simulink model "rocket"  (R2024a)
settings: Solver=ode5  StartTime=0.0  StopTime=time  FixedStep=0.01  RelTol=1e-3
values from neighbouring files (symbols this model uses):
  angle_ref = 0    [main.m]
  dt = 4    [main.m]
  F_side_thruster = 440    [main.m]
  F_thruster = 111000    [main.m]
  g = 9.81    [main.m]
  height = 8.15    [main.m]
  J = 1/12*m *(height^2 + 3*radius^2)    (= 4215.95433333)    [main.m]
  k = 0.02    [main.m]
  Ka = 1    [main.m]
  Kd = 0    [main.m]
  Ki = 0    [main.m]
  Kp = 0    [main.m]
  m = 760    [main.m]
  radius = 0.22    [main.m]
undefined symbols (not defined in the file or in its folder): W
settings Model: Creator=erlin  LastModifiedBy=erlin

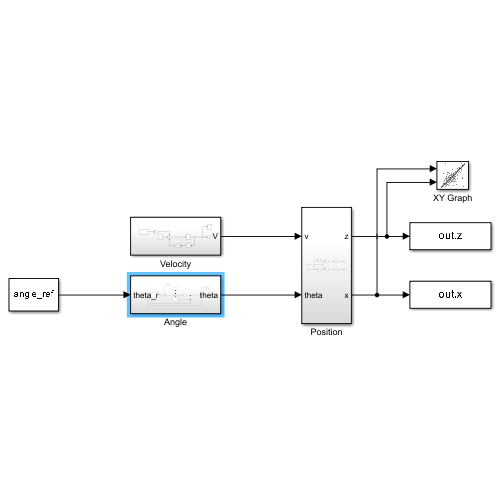
[thumbnail: Simulink's stored preview of the top-level diagram]
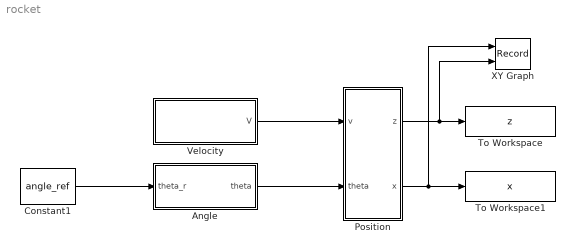
== system rocket ==
  Angle : Subsystem
  Constant1 : Constant  Value=angle_ref
  Position : Subsystem
  To Workspace : ToWorkspace  VariableName=z  SaveFormat=Timeseries  SampleTime=-1
  To Workspace1 : ToWorkspace  VariableName=x  SaveFormat=Timeseries  SampleTime=-1
  Velocity : Subsystem
  XY Graph : Record  FileSettingsInternal="{\"entries\":[{\"content\":{\"excelSettings\":{\"content\":{},\"type\":\"Streamout.ExcelSettings\"}},\"type\":\"Streamout.FileSettingStorage\",\"uuid\":\"\"}],\"packageUris\":[\"http:\\/\\/schema.mathworks.com\\/mf0\\/streamout_blocks\\/R2020a\"],\"version\":\"1.0\"}"  Layout=[1 1]  SignalsInternal="{\"entries\":[{\"content\":{\"signals\":[{\"content\":{\"blockPath\":[],\"dimensions\":[1],\"domain\":\"\",\"lineColor\":\"#a2142f\",\"plots\":[ 1 ],\"port\":1,\"sid\":[\"\"],\"signalID\":1,\"signalName\":\"Position:2\"},\"type\":\"RecordBlkView.Signal\",\"uuid\":\"\"},{\"content\":{\"blockPath\":[],\"dimensions\":[1],\"domain\":\"\",\"lineColor\":\"#139fff\",\"plots\":[ 1 ],\"port\":2,\"sid\":[\"\"],\"signalID\":2,\"signalName\":\"Position:1\"},\"type\":\"RecordBlkView.Signal\",\"uuid\":\"\"}]},\"type\":\"RecordBlkView.InputSignals\",\"uuid\":\"\"}],\"packageUris\":[\"http:\\/\\/schema.mathworks.com\\/mf0\\/streamout_blocks\\/R2020a\"],\"version\":\"1.0\"}"  VisualizationBindings="{\"xyplotplugin\":{\"info\":[{\"series\":[{\"bindingParametersList\":[{\"parameter\":\"X-Axis\",\"signalID\":1,\"signalName\":\"Position:2\"},{\"parameter\":\"Y-Axis\",\"signalID\":2,\"signalName\":\"Position:1\"}],\"seriesID\":0}],\"subplotID\":1}]}}"  CompatibilityTag=XY
  wires:
  Velocity/1(V) -> Position/1(v)
  Angle/1(theta) -> Position/2(theta)
  Position/1(z) -> XY Graph/2, To Workspace/1
  Position/2(x) -> XY Graph/1, To Workspace1/1
  Constant1/1 -> Angle/1(theta_r)

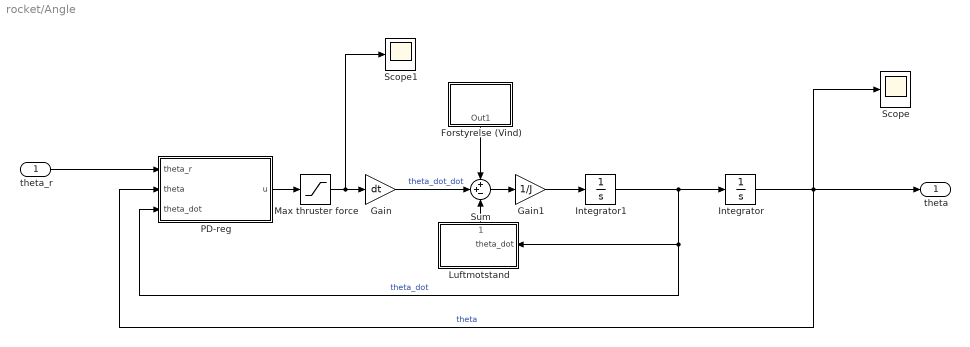
== system rocket/Angle ==
  theta_r : Inport
  Forstyrelse (Vind) : Subsystem
  Gain : Gain  Gain=dt
  Gain1 : Gain  Gain=1/J
  Integrator : Integrator
  Integrator1 : Integrator
  Luftmotstand : Subsystem
      settings: PortSchema="{\"entries\":[{\"content\":{\"sides\":[{\"content\":{},\"type\":\"ConnectorPlacement.EquallySpacedRectSide\",\"uuid\":\"0698149c-fc66-40d5-96ad-7619179b653e\"},{\"content\":{\"connectorIds\":[\"Out1\"],\"side\":\"RIGHT\"},\"type\":\"ConnectorPlacement.EquallySpacedRectSide\",\"uuid\":\"7770e965-7410-4cbf-a102-79b4cde0d90a\"},{\"content\":{\"side\":\"TOP\"},\"type\":\"ConnectorPlacement.EquallySpacedRectSide\",\"uuid\":\"2756d427-3d7a-4b20-bd26-ca223827eea1\"},{\"content\":{\"connectorIds\":[\"In1\"],\"side\":\"BOTTOM\"},\"type\":\"ConnectorPlacement.EquallySpacedRectSide\",\"uuid\":\"1c0a4e01-980e-4eae-bcaf-d8b95709db4d\"}]},\"type\":\"ConnectorPlacement.EquallySpacedConnector\",\"uuid\":\"871502e0-b275-4b38-8496-5b51979ecd95\"}],\"packageUris\":[\"http://schema.mathworks.com/mf0/Connector/R2020b\"],\"version\":\"1.0\"}"
  Max thruster force : Saturate  UpperLimit=F_side_thruster  LowerLimit=-F_side_thruster
  PD-reg : Subsystem
  Scope : Scope
  Scope1 : Scope
  Sum : Sum  Inputs=++-
  theta : Outport
  wires:
  Integrator1/1 -> Integrator/1, PD-reg/3(theta_dot), Luftmotstand/1(theta_dot)  "theta_dot"
  Integrator/1 -> PD-reg/2(theta), theta/1, Scope/1  "theta"
  Sum/1 -> Gain1/1
  Gain/1 -> Sum/2  "theta_dot_dot"
  theta_r/1 -> PD-reg/1(theta_r)
  Forstyrelse (Vind)/1(Out1) -> Sum/1
  PD-reg/1(u) -> Max thruster force/1
  Luftmotstand/1(1) -> Sum/3
  Gain1/1 -> Integrator1/1
  Max thruster force/1 -> Scope1/1, Gain/1

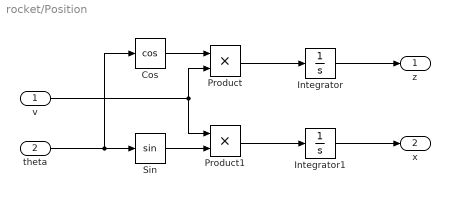
== system rocket/Position ==
  v : Inport
  theta : Inport  Port=2
  Cos : Trigonometry  Operator=cos
  Integrator : Integrator
  Integrator1 : Integrator
  Product : Product
  Product1 : Product
  Sin : Trigonometry
  z : Outport
  x : Outport  Port=2
  wires:
  theta/1 -> Cos/1, Sin/1
  v/1 -> Product1/1, Product/2
  Product/1 -> Integrator/1
  Product1/1 -> Integrator1/1
  Sin/1 -> Product1/2
  Integrator/1 -> z/1
  Integrator1/1 -> x/1
  Cos/1 -> Product/1

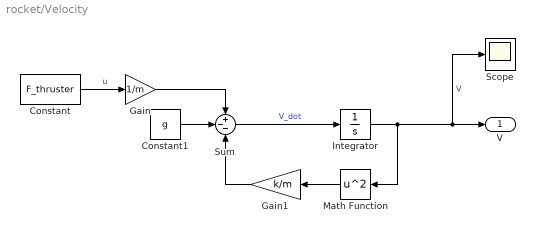
== system rocket/Velocity ==
  Constant : Constant  Value=F_thruster
  Constant1 : Constant  Value=g
  Gain : Gain  Gain=1/m
  Gain1 : Gain  Gain=k/m
  Integrator : Integrator
  Math Function : Math  Operator=square
  Scope : Scope
  Sum : Sum  Inputs=+--
  V : Outport
  wires:
  Constant1/1 -> Sum/2
  Gain/1 -> Sum/1
  Gain1/1 -> Sum/3
  Constant/1 -> Gain/1  "u"
  Integrator/1 -> Math Function/1, Scope/1, V/1  "V"
  Math Function/1 -> Gain1/1
  Sum/1 -> Integrator/1  "V_dot"

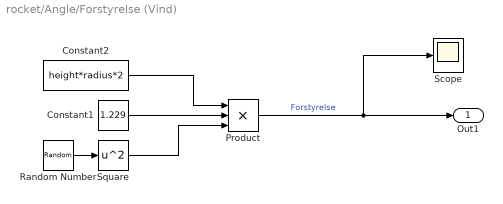
== system rocket/Angle/Forstyrelse (Vind) ==
  Constant1 : Constant  Value=1.229
  Constant2 : Constant  Value=height*radius*2
  Product : Product  Inputs=3
  Random Number : RandomNumber  Mean=W  Variance=W/2  SampleTime=10
  Scope : Scope
  Square : Math  Operator=square
  Out1 : Outport
  wires:
  Product/1 -> Scope/1, Out1/1  "Forstyrelse"
  Constant1/1 -> Product/2
  Constant2/1 -> Product/1
  Random Number/1 -> Square/1
  Square/1 -> Product/3

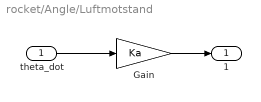
== system rocket/Angle/Luftmotstand ==
  theta_dot : Inport
  Gain : Gain  Gain=Ka
  1 : Outport
  wires:
  Gain/1 -> 1/1
  theta_dot/1 -> Gain/1

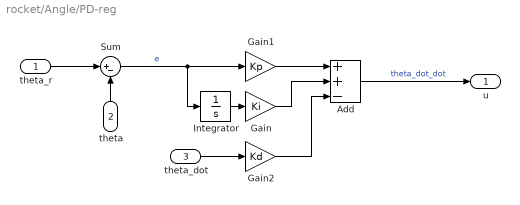
== system rocket/Angle/PD-reg ==
  theta_r : Inport
  theta : Inport  Port=2
  theta_dot : Inport  Port=3
  Add : Sum  Inputs=++-
  Gain : Gain  Gain=Ki
  Gain1 : Gain  Gain=Kp
  Gain2 : Gain  Gain=Kd
  Integrator : Integrator
  Sum : Sum  Inputs=|+-
  u : Outport
  wires:
  Gain2/1 -> Add/3
  Gain1/1 -> Add/1
  Sum/1 -> Integrator/1, Gain1/1  "e"
  Add/1 -> u/1  "theta_dot_dot"
  theta_r/1 -> Sum/1
  theta/1 -> Sum/2
  theta_dot/1 -> Gain2/1
  Integrator/1 -> Gain/1
  Gain/1 -> Add/2
